simulink model "L3closedloop"  (R2023b)
settings: Solver=VariableStepAuto  StartTime=0.0  StopTime=50.0  RelTol=1e-3
settings Model: Creator=Prince singh  LastModifiedBy=Prince singh

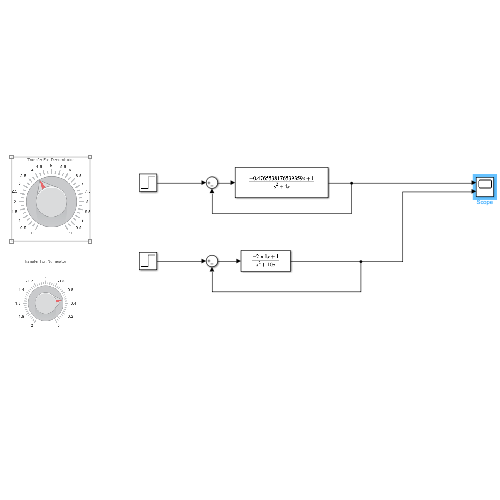
[thumbnail: Simulink's stored preview of the top-level diagram]
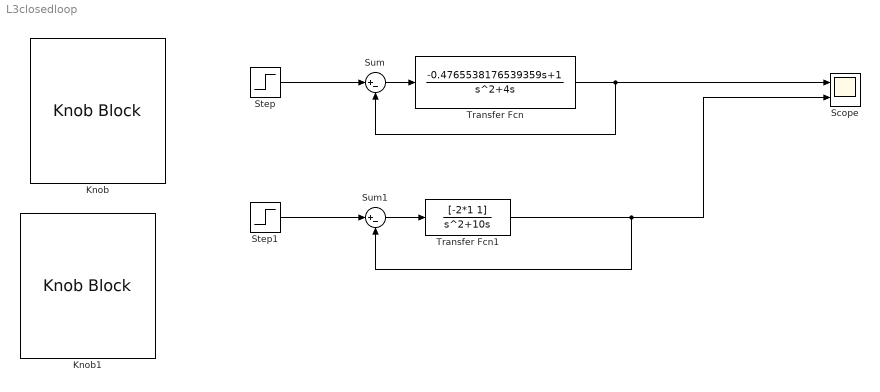
== system L3closedloop ==
  Knob : KnobBlock  ScaleMax=10
  Knob1 : KnobBlock  ScaleMin=-2  ScaleMax=0
  Scope : Scope  NumInputPorts=2
  Step : Step  SampleTime=0
  Step1 : Step  SampleTime=0
  Sum : Sum  Inputs=|+-
  Sum1 : Sum  Inputs=|+-
  Transfer Fcn : TransferFcn  Numerator=[-0.4765538176539359,1]  Denominator=[1,4,0]
  Transfer Fcn1 : TransferFcn  Numerator=[-2*1 1]  Denominator=[1 10 0]
  wires:
  Sum/1 -> Transfer Fcn/1
  Transfer Fcn/1 -> Sum/2, Scope/1
  Step/1 -> Sum/1
  Step1/1 -> Sum1/1
  Sum1/1 -> Transfer Fcn1/1
  Transfer Fcn1/1 -> Sum1/2, Scope/2
